simulink model "model01_limited"  (Simulink 7.9)
settings: Solver=ode45  StartTime=0.0  StopTime=10.0  RelTol=1e-3
undefined symbols (not defined in the file): initE, Kp, T
settings Model: Creator=ex16  LastModifiedBy=ex16

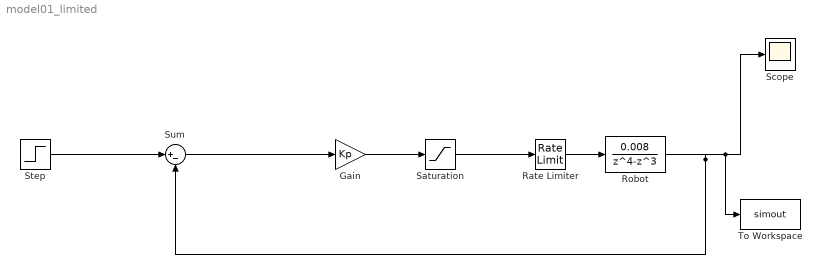
== system model01_limited ==
  Gain : Gain  Gain=Kp  SampleTime=T
  Rate Limiter : RateLimiter  RisingSlewLimit=15  FallingSlewLimit=-15  SampleTimeMode=inherited
  Robot : DiscreteTransferFcn  Numerator=[0.008]  Denominator=[1 -1 0 0 0]  SampleTime=T
  Saturation : Saturate  UpperLimit=3.2  LowerLimit=-3.2  SampleTime=T
  Scope : Scope
  Step : Step  Time=0  After=initE  SampleTime=T
  Sum : Sum  Inputs=|+-
  To Workspace : ToWorkspace  VariableName=simout  SampleTime=-1  SaveFormat=Structure With Time
  wires:
  Gain/1 -> Saturation/1
  Sum/1 -> Gain/1
  Robot/1 -> Sum/2, To Workspace/1, Scope/1
  Step/1 -> Sum/1
  Saturation/1 -> Rate Limiter/1
  Rate Limiter/1 -> Robot/1
